simulink model "Lab_Five_QRD_Other_Input"  (R2021a)
settings: Solver=VariableStepAuto  StartTime=0.0  StopTime=double(sim_length)  RelTol=1e-3
libraries: hdlBasic x61, hdlSSR x2, xbsIndex_r4 x1
settings Model: Creator=ckk5  LastModifiedBy=ckk5

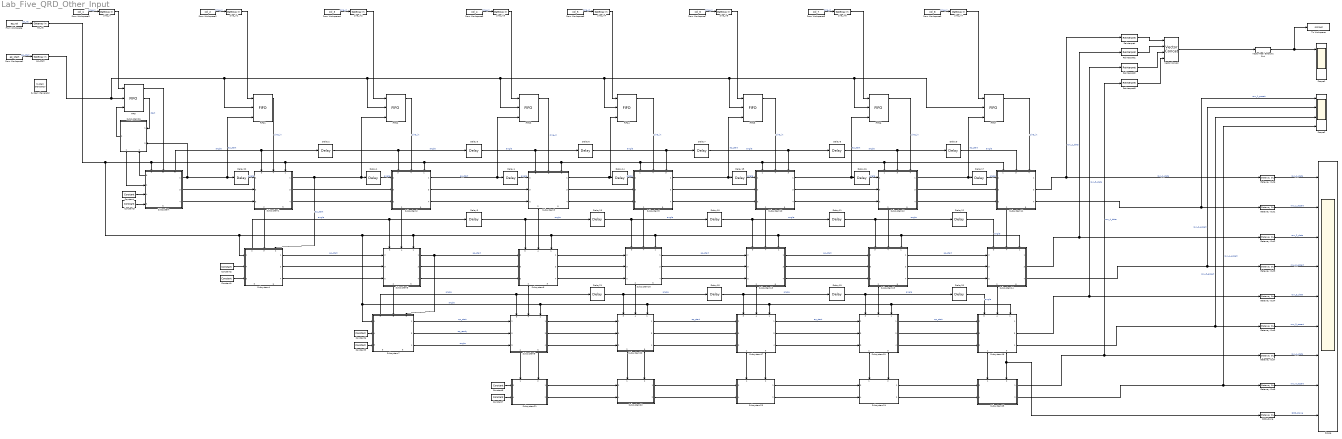
== system Lab_Five_QRD_Other_Input ==
  " System Generator" : xbsIndex_r4/ System Generator  Tag=genX  xilinxfamily=zynq  part=xc7z020  speed=-1  package=clg484  synthesis_tool=Vivado  clock_wrapper=Clock Enables  directory=./netlist  proj_type=Vivado  Synth_file=Vivado Synthesis Defaults  Impl_file=Vivado Implementation Defaults  testbench=off  simulink_period=1  sysclk_period=10  dcm_input_clock_period=10  incr_netlist=off  trim_vbits=Everywhere in SubSystem  dbl_ovrd=According to Block Masks  core_generation=According to Block Masks  run_coregen=off  deprecated_control=off  eval_field=0  block_type=sysgen
  Constant{,2,6,8} (4 alike) : hdlBasic/Constant  const=0  gui_display_data_type=Fixed-point  arith_type=Signed (2's comp)  n_bits=16  bin_pt=12  preci_type=Single  exp_width=8  frac_width=24  explicit_period=off  period=1  XmcBlockStatus=1  maskContainerNames=tabcontainer1  block_type=constant  block_config=sysgen:Constant_config
  Constant1 : hdlBasic/Constant  const=0  gui_display_data_type=Boolean  arith_type=Boolean  n_bits=16  bin_pt=12  preci_type=Single  exp_width=8  frac_width=24  explicit_period=off  period=1  XmcBlockStatus=1  maskContainerNames=tabcontainer1  block_type=constant  block_config=sysgen:Constant_config
  Constant3 : hdlBasic/Constant  const=0  gui_display_data_type=Boolean  arith_type=Boolean  n_bits=16  bin_pt=14  preci_type=Single  exp_width=8  frac_width=24  explicit_period=off  period=1  XmcBlockStatus=1  maskContainerNames=tabcontainer1  block_type=constant  block_config=sysgen:Constant_config
  Constant5 : hdlBasic/Constant  const=0  gui_display_data_type=Boolean  arith_type=Boolean  n_bits=16  bin_pt=12  preci_type=Single  exp_width=8  frac_width=24  explicit_period=off  period=1  XmcBlockStatus=1  maskContainerNames=tabcontainer1  block_type=constant  block_config=sysgen:Constant_config
  Constant7 : hdlBasic/Constant  const=0  gui_display_data_type=Boolean  arith_type=Boolean  n_bits=16  bin_pt=12  preci_type=Single  exp_width=8  frac_width=24  explicit_period=off  period=1  XmcBlockStatus=1  maskContainerNames=tabcontainer1  block_type=constant  block_config=sysgen:Constant_config
  Delay{1,4,14..17,22} (7 alike) : hdlBasic/Delay  rst=off  en=off  latency=1  reg_retiming=off  XmcBlockStatus=1  maskContainerNames=group1  block_type=delay  block_config=sysgen:Delay_config
  Delay{2..3,5..13,18..21} (15 alike) : hdlBasic/Delay  rst=off  en=off  latency=unit_L  reg_retiming=off  XmcBlockStatus=1  maskContainerNames=group1  block_type=delay  block_config=sysgen:Delay_config
  FIFO{,1..7} (8 alike) : hdlBasic/FIFO  mem_type=Block RAM  performance_options=Standard_FIFO  embedded_registers=off  depth=16  use_asym_data_widths=off  asym_read_width=32  percent_nbits=1  rst=off  rst_latency=1  en=off  use_dcount=off  use_percent_full_port=off  use_almost_empty=off  almost_empty_thresh=2  use_almost_full=off  use_rd_rst_busy=off  use_wr_rst_busy=off  almost_full_thresh=13  almost_empty_offset=[]  almost_full_offset=[]  explicit_period=off  period=[]  store_only_valid=[]  init_zero=[]  simulation_type=fast_sim  XmcBlockStatus=1  maskContainerNames=tabcontainer1  block_type=fifo  block_config=sysgen:FIFO_config
      settings: infoedit=[]
  From Workspace : FromWorkspace  VariableName=ap_rst
  From Workspace1 : FromWorkspace  VariableName=ap_start  OutputAfterFinalValue=Holding final value
  From Workspace2 : FromWorkspace  VariableName=col_2
  From Workspace3 : FromWorkspace  VariableName=col_1  OutputAfterFinalValue=Holding final value
  From Workspace4 : FromWorkspace  VariableName=col_3
  From Workspace5 : FromWorkspace  VariableName=col_4
  From Workspace6 : FromWorkspace  VariableName=col_5
  From Workspace7 : FromWorkspace  VariableName=col_6
  From Workspace8 : FromWorkspace  VariableName=col_7
  From Workspace9 : FromWorkspace  VariableName=col_8
  Gateway Out{1..8} (8 alike) : hdlBasic/Gateway Out  inherit_from_input=off  hdl_port=on  rows=1  columns=1  UseAsDAC=off  DACChannel='1'  interface=None  automatic_assignment=on  address_offset=hex2dec('00')  intf_name=''  intf_description=''  timing_constraint=None  locs_specified=off  LOCs={}  io_standard={}  XmcBlockStatus=1  maskContainerNames=group4  block_type=gatewayout  block_config=sysgen:gateway_out_config  block_width_w=590  block_height_w=620  block_width=620  block_height=750
  QRD_Done : hdlBasic/Gateway Out  inherit_from_input=off  hdl_port=on  rows=1  columns=1  UseAsDAC=off  DACChannel='1'  interface=None  automatic_assignment=on  address_offset=hex2dec('00')  intf_name=''  intf_description=''  timing_constraint=None  locs_specified=off  LOCs={}  io_standard={}  XmcBlockStatus=1  maskContainerNames=group4  block_type=gatewayout  block_config=sysgen:gateway_out_config  block_width_w=590  block_height_w=620  block_width=620  block_height=750
  Reinterpret{,1..3} (4 alike) : hdlBasic/Reinterpret  force_arith_type=on  arith_type=Unsigned  force_bin_pt=on  bin_pt=0  XmcBlockStatus=1  maskContainerNames=group1  block_type=reinterpret  block_config=sysgen:Reinterpret_config
  Scope : Scope  NumInputPorts=9
  Scope1 : Scope  NumInputPorts=3
  Scope2 : Scope  NumInputPorts=4
  Subsystem : Subsystem  ReferencedSubsystem=ATAN
      settings: PortSchema="{\"entries\":[{\"content\":{\"sides\":[{\"content\":{\"connectorIds\":[\"Out6\",\"In2\",\"In4\",\"In5\"]},\"type\":\"ConnectorPlacement.EquallySpacedRectSide\",\"uuid\":\"1346c518-8b2f-4526-a2ea-39cbeadf4b85\"},{\"content\":{\"connectorIds\":[\"Out1\",\"Out3\",\"Out4\"],\"side\":\"RIGHT\"},\"type\":\"ConnectorPlacement.EquallySpacedRectSide\",\"uuid\":\"7c1b3206-bde6-4225-9c16-bfac1b31b1ce\"},{\"content\":{\"connectorIds\":[\"In1\",\"In3\",\"Out2\"],\"side\":\"TOP\"},\"type\":\"ConnectorPlacement.EquallySpacedRectSide\",\"uuid\":\"34800851-84f6-4615-adc5-1b8c9e241528\"},{\"content\":{\"connectorIds\":[\"Out5\"],\"side\":\"BOTTOM\"},\"type\":\"ConnectorPlacement.EquallySpacedRectSide\",\"uuid\":\"52413a32-a386-4ce7-b0e4-3384f003f446\"}]},\"type\":\"ConnectorPlacement.EquallySpacedConnector\",\"uuid\":\"4bca380c-1fcc-49d9-b3a4-0ea90ddd08bc\"}],\"packageUris\":[\"http://schema.mathworks.com/mf0/Connector/R2020b\"],\"version\":\"1.0\"}"
  Subsystem{1..3,5..6,8..20} (18 alike) : Subsystem  ReferencedSubsystem=ROT
      Subsystem1 settings: PortSchema="{\"entries\":[{\"content\":{\"sides\":[{\"content\":{\"connectorIds\":[\"In2\",\"In5\",\"In6\"]},\"type\":\"ConnectorPlacement.EquallySpacedRectSide\",\"uuid\":\"c545b77a-6185-4f00-b3c2-6f0e95b73481\"},{\"content\":{\"connectorIds\":[\"Out1\",\"Out3\",\"Out4\"],\"side\":\"RIGHT\"},\"type\":\"ConnectorPlacement.EquallySpacedRectSide\",\"uuid\":\"77b30f40-c5e6-4fc5-a8bf-3f587adee46d\"},{\"content\":{\"connectorIds\":[\"In3\",\"In4\",\"In1\"],\"side\":\"TOP\"},\"type\":\"ConnectorPlacement.EquallySpacedRectSide\",\"uuid\":\"0350c9e1-b4fb-456c-83bc-c0f4f7513119\"},{\"content\":{\"connectorIds\":[\"Out2\",\"Out5\"],\"side\":\"BOTTOM\"},\"type\":\"ConnectorPlacement.EquallySpacedRectSide\",\"uuid\":\"941caaa4-bb26-4816-a397-9ab84bd5a497\"}]},\"type\":\"ConnectorPlacement.EquallySpacedConnector\",\"uuid\":\"f70f627f-f2df-4c33-aee4-d408a53254f2\"}],\"packageUris\":[\"http://schema.mathworks.com/mf0/Connector/R2020b\"],\"version\":\"1.0\"}"
      Subsystem10 settings: PortSchema="{\"entries\":[{\"content\":{\"sides\":[{\"content\":{\"connectorIds\":[\"In2\",\"In5\",\"In6\"]},\"type\":\"ConnectorPlacement.EquallySpacedRectSide\",\"uuid\":\"c545b77a-6185-4f00-b3c2-6f0e95b73481\"},{\"content\":{\"connectorIds\":[\"Out1\",\"Out3\",\"Out4\"],\"side\":\"RIGHT\"},\"type\":\"ConnectorPlacement.EquallySpacedRectSide\",\"uuid\":\"77b30f40-c5e6-4fc5-a8bf-3f587adee46d\"},{\"content\":{\"connectorIds\":[\"In1\",\"In4\",\"In3\"],\"side\":\"TOP\"},\"type\":\"ConnectorPlacement.EquallySpacedRectSide\",\"uuid\":\"0350c9e1-b4fb-456c-83bc-c0f4f7513119\"},{\"content\":{\"connectorIds\":[\"Out2\",\"Out5\"],\"side\":\"BOTTOM\"},\"type\":\"ConnectorPlacement.EquallySpacedRectSide\",\"uuid\":\"762d5bef-bc89-4a37-a25e-dba0fd023964\"}]},\"type\":\"ConnectorPlacement.EquallySpacedConnector\",\"uuid\":\"f70f627f-f2df-4c33-aee4-d408a53254f2\"}],\"packageUris\":[\"http://schema.mathworks.com/mf0/Connector/R2020b\"],\"version\":\"1.0\"}"
      Subsystem11 settings: PortSchema="{\"entries\":[{\"content\":{\"sides\":[{\"content\":{\"connectorIds\":[\"In2\",\"In5\",\"In6\"]},\"type\":\"ConnectorPlacement.EquallySpacedRectSide\",\"uuid\":\"c545b77a-6185-4f00-b3c2-6f0e95b73481\"},{\"content\":{\"connectorIds\":[\"Out1\",\"Out3\",\"Out4\"],\"side\":\"RIGHT\"},\"type\":\"ConnectorPlacement.EquallySpacedRectSide\",\"uuid\":\"77b30f40-c5e6-4fc5-a8bf-3f587adee46d\"},{\"content\":{\"connectorIds\":[\"In1\",\"In3\",\"In4\"],\"side\":\"TOP\"},\"type\":\"ConnectorPlacement.EquallySpacedRectSide\",\"uuid\":\"0350c9e1-b4fb-456c-83bc-c0f4f7513119\"},{\"content\":{\"connectorIds\":[\"Out2\",\"Out5\"],\"side\":\"BOTTOM\"},\"type\":\"ConnectorPlacement.EquallySpacedRectSide\",\"uuid\":\"5cdcca09-d0a6-4fbe-ad32-f85ef7564229\"}]},\"type\":\"ConnectorPlacement.EquallySpacedConnector\",\"uuid\":\"f70f627f-f2df-4c33-aee4-d408a53254f2\"}],\"packageUris\":[\"http://schema.mathworks.com/mf0/Connector/R2020b\"],\"version\":\"1.0\"}"
      Subsystem12 settings: PortSchema="{\"entries\":[{\"content\":{\"sides\":[{\"content\":{\"connectorIds\":[\"In2\",\"In5\",\"In6\"]},\"type\":\"ConnectorPlacement.EquallySpacedRectSide\",\"uuid\":\"c545b77a-6185-4f00-b3c2-6f0e95b73481\"},{\"content\":{\"connectorIds\":[\"Out1\",\"Out3\",\"Out4\"],\"side\":\"RIGHT\"},\"type\":\"ConnectorPlacement.EquallySpacedRectSide\",\"uuid\":\"77b30f40-c5e6-4fc5-a8bf-3f587adee46d\"},{\"content\":{\"connectorIds\":[\"In1\",\"In3\",\"In4\"],\"side\":\"TOP\"},\"type\":\"ConnectorPlacement.EquallySpacedRectSide\",\"uuid\":\"0350c9e1-b4fb-456c-83bc-c0f4f7513119\"},{\"content\":{\"connectorIds\":[\"Out2\",\"Out5\"],\"side\":\"BOTTOM\"},\"type\":\"ConnectorPlacement.EquallySpacedRectSide\",\"uuid\":\"eee39a82-822b-43a0-8e38-2b49c729ce24\"}]},\"type\":\"ConnectorPlacement.EquallySpacedConnector\",\"uuid\":\"f70f627f-f2df-4c33-aee4-d408a53254f2\"}],\"packageUris\":[\"http://schema.mathworks.com/mf0/Connector/R2020b\"],\"version\":\"1.0\"}"
      Subsystem13 settings: PortSchema="{\"entries\":[{\"content\":{\"sides\":[{\"content\":{\"connectorIds\":[\"In2\",\"In5\",\"In6\"]},\"type\":\"ConnectorPlacement.EquallySpacedRectSide\",\"uuid\":\"c545b77a-6185-4f00-b3c2-6f0e95b73481\"},{\"content\":{\"connectorIds\":[\"Out1\",\"Out3\",\"Out4\"],\"side\":\"RIGHT\"},\"type\":\"ConnectorPlacement.EquallySpacedRectSide\",\"uuid\":\"77b30f40-c5e6-4fc5-a8bf-3f587adee46d\"},{\"content\":{\"connectorIds\":[\"In3\",\"In4\",\"In1\"],\"side\":\"TOP\"},\"type\":\"ConnectorPlacement.EquallySpacedRectSide\",\"uuid\":\"0350c9e1-b4fb-456c-83bc-c0f4f7513119\"},{\"content\":{\"connectorIds\":[\"Out2\",\"Out5\"],\"side\":\"BOTTOM\"},\"type\":\"ConnectorPlacement.EquallySpacedRectSide\",\"uuid\":\"123044bf-0605-4816-88b3-d54ecb8af519\"}]},\"type\":\"ConnectorPlacement.EquallySpacedConnector\",\"uuid\":\"f70f627f-f2df-4c33-aee4-d408a53254f2\"}],\"packageUris\":[\"http://schema.mathworks.com/mf0/Connector/R2020b\"],\"version\":\"1.0\"}"
      Subsystem14 settings: PortSchema="{\"entries\":[{\"content\":{\"sides\":[{\"content\":{\"connectorIds\":[\"In2\",\"In5\",\"In6\"]},\"type\":\"ConnectorPlacement.EquallySpacedRectSide\",\"uuid\":\"c545b77a-6185-4f00-b3c2-6f0e95b73481\"},{\"content\":{\"connectorIds\":[\"Out1\",\"Out3\",\"Out4\"],\"side\":\"RIGHT\"},\"type\":\"ConnectorPlacement.EquallySpacedRectSide\",\"uuid\":\"77b30f40-c5e6-4fc5-a8bf-3f587adee46d\"},{\"content\":{\"connectorIds\":[\"In3\",\"In4\",\"In1\"],\"side\":\"TOP\"},\"type\":\"ConnectorPlacement.EquallySpacedRectSide\",\"uuid\":\"0350c9e1-b4fb-456c-83bc-c0f4f7513119\"},{\"content\":{\"connectorIds\":[\"Out2\",\"Out5\"],\"side\":\"BOTTOM\"},\"type\":\"ConnectorPlacement.EquallySpacedRectSide\",\"uuid\":\"c378bf0f-4acf-4a5e-92e8-43e03dc0127f\"}]},\"type\":\"ConnectorPlacement.EquallySpacedConnector\",\"uuid\":\"f70f627f-f2df-4c33-aee4-d408a53254f2\"}],\"packageUris\":[\"http://schema.mathworks.com/mf0/Connector/R2020b\"],\"version\":\"1.0\"}"
      Subsystem15 settings: PortSchema="{\"entries\":[{\"content\":{\"sides\":[{\"content\":{\"connectorIds\":[\"In2\",\"In5\",\"In6\"]},\"type\":\"ConnectorPlacement.EquallySpacedRectSide\",\"uuid\":\"c545b77a-6185-4f00-b3c2-6f0e95b73481\"},{\"content\":{\"connectorIds\":[\"Out1\",\"Out3\",\"Out4\"],\"side\":\"RIGHT\"},\"type\":\"ConnectorPlacement.EquallySpacedRectSide\",\"uuid\":\"77b30f40-c5e6-4fc5-a8bf-3f587adee46d\"},{\"content\":{\"connectorIds\":[\"In3\",\"In4\",\"In1\"],\"side\":\"TOP\"},\"type\":\"ConnectorPlacement.EquallySpacedRectSide\",\"uuid\":\"0350c9e1-b4fb-456c-83bc-c0f4f7513119\"},{\"content\":{\"connectorIds\":[\"Out2\",\"Out5\"],\"side\":\"BOTTOM\"},\"type\":\"ConnectorPlacement.EquallySpacedRectSide\",\"uuid\":\"d7dbbe88-442b-4e14-87a2-1b50104b2bcd\"}]},\"type\":\"ConnectorPlacement.EquallySpacedConnector\",\"uuid\":\"f70f627f-f2df-4c33-aee4-d408a53254f2\"}],\"packageUris\":[\"http://schema.mathworks.com/mf0/Connector/R2020b\"],\"version\":\"1.0\"}"
      Subsystem16 settings: PortSchema="{\"entries\":[{\"content\":{\"sides\":[{\"content\":{\"connectorIds\":[\"In2\",\"In5\",\"In6\"]},\"type\":\"ConnectorPlacement.EquallySpacedRectSide\",\"uuid\":\"c545b77a-6185-4f00-b3c2-6f0e95b73481\"},{\"content\":{\"connectorIds\":[\"Out1\",\"Out3\",\"Out4\"],\"side\":\"RIGHT\"},\"type\":\"ConnectorPlacement.EquallySpacedRectSide\",\"uuid\":\"77b30f40-c5e6-4fc5-a8bf-3f587adee46d\"},{\"content\":{\"connectorIds\":[\"In3\",\"In4\",\"In1\"],\"side\":\"TOP\"},\"type\":\"ConnectorPlacement.EquallySpacedRectSide\",\"uuid\":\"0350c9e1-b4fb-456c-83bc-c0f4f7513119\"},{\"content\":{\"connectorIds\":[\"Out2\",\"Out5\"],\"side\":\"BOTTOM\"},\"type\":\"ConnectorPlacement.EquallySpacedRectSide\",\"uuid\":\"9556fa50-b1e5-4995-ad98-fda291ad635e\"}]},\"type\":\"ConnectorPlacement.EquallySpacedConnector\",\"uuid\":\"f70f627f-f2df-4c33-aee4-d408a53254f2\"}],\"packageUris\":[\"http://schema.mathworks.com/mf0/Connector/R2020b\"],\"version\":\"1.0\"}"
      Subsystem17 settings: PortSchema="{\"entries\":[{\"content\":{\"sides\":[{\"content\":{\"connectorIds\":[\"In2\",\"In5\",\"In6\"]},\"type\":\"ConnectorPlacement.EquallySpacedRectSide\",\"uuid\":\"c545b77a-6185-4f00-b3c2-6f0e95b73481\"},{\"content\":{\"connectorIds\":[\"Out1\",\"Out3\",\"Out4\"],\"side\":\"RIGHT\"},\"type\":\"ConnectorPlacement.EquallySpacedRectSide\",\"uuid\":\"77b30f40-c5e6-4fc5-a8bf-3f587adee46d\"},{\"content\":{\"connectorIds\":[\"In3\",\"In4\",\"In1\"],\"side\":\"TOP\"},\"type\":\"ConnectorPlacement.EquallySpacedRectSide\",\"uuid\":\"0350c9e1-b4fb-456c-83bc-c0f4f7513119\"},{\"content\":{\"connectorIds\":[\"Out2\",\"Out5\"],\"side\":\"BOTTOM\"},\"type\":\"ConnectorPlacement.EquallySpacedRectSide\",\"uuid\":\"123044bf-0605-4816-88b3-d54ecb8af519\"}]},\"type\":\"ConnectorPlacement.EquallySpacedConnector\",\"uuid\":\"f70f627f-f2df-4c33-aee4-d408a53254f2\"}],\"packageUris\":[\"http://schema.mathworks.com/mf0/Connector/R2020b\"],\"version\":\"1.0\"}"
      Subsystem18 settings: PortSchema="{\"entries\":[{\"content\":{\"sides\":[{\"content\":{\"connectorIds\":[\"In2\",\"In5\",\"In6\"]},\"type\":\"ConnectorPlacement.EquallySpacedRectSide\",\"uuid\":\"c545b77a-6185-4f00-b3c2-6f0e95b73481\"},{\"content\":{\"connectorIds\":[\"Out1\",\"Out3\",\"Out4\"],\"side\":\"RIGHT\"},\"type\":\"ConnectorPlacement.EquallySpacedRectSide\",\"uuid\":\"77b30f40-c5e6-4fc5-a8bf-3f587adee46d\"},{\"content\":{\"connectorIds\":[\"In3\",\"In4\",\"In1\"],\"side\":\"TOP\"},\"type\":\"ConnectorPlacement.EquallySpacedRectSide\",\"uuid\":\"0350c9e1-b4fb-456c-83bc-c0f4f7513119\"},{\"content\":{\"connectorIds\":[\"Out2\",\"Out5\"],\"side\":\"BOTTOM\"},\"type\":\"ConnectorPlacement.EquallySpacedRectSide\",\"uuid\":\"d882beaa-ab78-4a12-aee9-70b010452786\"}]},\"type\":\"ConnectorPlacement.EquallySpacedConnector\",\"uuid\":\"f70f627f-f2df-4c33-aee4-d408a53254f2\"}],\"packageUris\":[\"http://schema.mathworks.com/mf0/Connector/R2020b\"],\"version\":\"1.0\"}"
      Subsystem19 settings: PortSchema="{\"entries\":[{\"content\":{\"sides\":[{\"content\":{\"connectorIds\":[\"In2\",\"In5\",\"In6\"]},\"type\":\"ConnectorPlacement.EquallySpacedRectSide\",\"uuid\":\"c545b77a-6185-4f00-b3c2-6f0e95b73481\"},{\"content\":{\"connectorIds\":[\"Out1\",\"Out3\",\"Out4\"],\"side\":\"RIGHT\"},\"type\":\"ConnectorPlacement.EquallySpacedRectSide\",\"uuid\":\"77b30f40-c5e6-4fc5-a8bf-3f587adee46d\"},{\"content\":{\"connectorIds\":[\"In3\",\"In4\",\"In1\"],\"side\":\"TOP\"},\"type\":\"ConnectorPlacement.EquallySpacedRectSide\",\"uuid\":\"0350c9e1-b4fb-456c-83bc-c0f4f7513119\"},{\"content\":{\"connectorIds\":[\"Out2\",\"Out5\"],\"side\":\"BOTTOM\"},\"type\":\"ConnectorPlacement.EquallySpacedRectSide\",\"uuid\":\"d7dbbe88-442b-4e14-87a2-1b50104b2bcd\"}]},\"type\":\"ConnectorPlacement.EquallySpacedConnector\",\"uuid\":\"f70f627f-f2df-4c33-aee4-d408a53254f2\"}],\"packageUris\":[\"http://schema.mathworks.com/mf0/Connector/R2020b\"],\"version\":\"1.0\"}"
      Subsystem2 settings: PortSchema="{\"entries\":[{\"content\":{\"sides\":[{\"content\":{\"connectorIds\":[\"In2\",\"In5\",\"In6\"]},\"type\":\"ConnectorPlacement.EquallySpacedRectSide\",\"uuid\":\"c545b77a-6185-4f00-b3c2-6f0e95b73481\"},{\"content\":{\"connectorIds\":[\"Out1\",\"Out3\",\"Out4\"],\"side\":\"RIGHT\"},\"type\":\"ConnectorPlacement.EquallySpacedRectSide\",\"uuid\":\"77b30f40-c5e6-4fc5-a8bf-3f587adee46d\"},{\"content\":{\"connectorIds\":[\"In3\",\"In4\",\"In1\"],\"side\":\"TOP\"},\"type\":\"ConnectorPlacement.EquallySpacedRectSide\",\"uuid\":\"0350c9e1-b4fb-456c-83bc-c0f4f7513119\"},{\"content\":{\"connectorIds\":[\"Out2\",\"Out5\"],\"side\":\"BOTTOM\"},\"type\":\"ConnectorPlacement.EquallySpacedRectSide\",\"uuid\":\"9359a6a3-4861-4aac-b9db-7dc0ab9ac5b9\"}]},\"type\":\"ConnectorPlacement.EquallySpacedConnector\",\"uuid\":\"f70f627f-f2df-4c33-aee4-d408a53254f2\"}],\"packageUris\":[\"http://schema.mathworks.com/mf0/Connector/R2020b\"],\"version\":\"1.0\"}"
      Subsystem20 settings: PortSchema="{\"entries\":[{\"content\":{\"sides\":[{\"content\":{\"connectorIds\":[\"In2\",\"In5\",\"In6\"]},\"type\":\"ConnectorPlacement.EquallySpacedRectSide\",\"uuid\":\"c545b77a-6185-4f00-b3c2-6f0e95b73481\"},{\"content\":{\"connectorIds\":[\"Out1\",\"Out3\",\"Out4\"],\"side\":\"RIGHT\"},\"type\":\"ConnectorPlacement.EquallySpacedRectSide\",\"uuid\":\"77b30f40-c5e6-4fc5-a8bf-3f587adee46d\"},{\"content\":{\"connectorIds\":[\"In3\",\"In4\",\"In1\"],\"side\":\"TOP\"},\"type\":\"ConnectorPlacement.EquallySpacedRectSide\",\"uuid\":\"0350c9e1-b4fb-456c-83bc-c0f4f7513119\"},{\"content\":{\"connectorIds\":[\"Out2\",\"Out5\"],\"side\":\"BOTTOM\"},\"type\":\"ConnectorPlacement.EquallySpacedRectSide\",\"uuid\":\"9556fa50-b1e5-4995-ad98-fda291ad635e\"}]},\"type\":\"ConnectorPlacement.EquallySpacedConnector\",\"uuid\":\"f70f627f-f2df-4c33-aee4-d408a53254f2\"}],\"packageUris\":[\"http://schema.mathworks.com/mf0/Connector/R2020b\"],\"version\":\"1.0\"}"
      Subsystem3 settings: PortSchema="{\"entries\":[{\"content\":{\"sides\":[{\"content\":{\"connectorIds\":[\"In2\",\"In5\",\"In6\"]},\"type\":\"ConnectorPlacement.EquallySpacedRectSide\",\"uuid\":\"c545b77a-6185-4f00-b3c2-6f0e95b73481\"},{\"content\":{\"connectorIds\":[\"Out1\",\"Out3\",\"Out4\"],\"side\":\"RIGHT\"},\"type\":\"ConnectorPlacement.EquallySpacedRectSide\",\"uuid\":\"77b30f40-c5e6-4fc5-a8bf-3f587adee46d\"},{\"content\":{\"connectorIds\":[\"In3\",\"In4\",\"In1\"],\"side\":\"TOP\"},\"type\":\"ConnectorPlacement.EquallySpacedRectSide\",\"uuid\":\"0350c9e1-b4fb-456c-83bc-c0f4f7513119\"},{\"content\":{\"connectorIds\":[\"Out2\",\"Out5\"],\"side\":\"BOTTOM\"},\"type\":\"ConnectorPlacement.EquallySpacedRectSide\",\"uuid\":\"8be21b47-252e-49f0-b877-01a730546064\"}]},\"type\":\"ConnectorPlacement.EquallySpacedConnector\",\"uuid\":\"f70f627f-f2df-4c33-aee4-d408a53254f2\"}],\"packageUris\":[\"http://schema.mathworks.com/mf0/Connector/R2020b\"],\"version\":\"1.0\"}"
      Subsystem5 settings: PortSchema="{\"entries\":[{\"content\":{\"sides\":[{\"content\":{\"connectorIds\":[\"In2\",\"In5\",\"In6\"]},\"type\":\"ConnectorPlacement.EquallySpacedRectSide\",\"uuid\":\"c545b77a-6185-4f00-b3c2-6f0e95b73481\"},{\"content\":{\"connectorIds\":[\"Out1\",\"Out3\",\"Out4\"],\"side\":\"RIGHT\"},\"type\":\"ConnectorPlacement.EquallySpacedRectSide\",\"uuid\":\"77b30f40-c5e6-4fc5-a8bf-3f587adee46d\"},{\"content\":{\"connectorIds\":[\"In3\",\"In4\",\"In1\"],\"side\":\"TOP\"},\"type\":\"ConnectorPlacement.EquallySpacedRectSide\",\"uuid\":\"0350c9e1-b4fb-456c-83bc-c0f4f7513119\"},{\"content\":{\"connectorIds\":[\"Out2\",\"Out5\"],\"side\":\"BOTTOM\"},\"type\":\"ConnectorPlacement.EquallySpacedRectSide\",\"uuid\":\"8ce605ee-a3e7-450c-b19e-841b4c6bf8e9\"}]},\"type\":\"ConnectorPlacement.EquallySpacedConnector\",\"uuid\":\"f70f627f-f2df-4c33-aee4-d408a53254f2\"}],\"packageUris\":[\"http://schema.mathworks.com/mf0/Connector/R2020b\"],\"version\":\"1.0\"}"
      Subsystem6 settings: PortSchema="{\"entries\":[{\"content\":{\"sides\":[{\"content\":{\"connectorIds\":[\"In2\",\"In5\",\"In6\"]},\"type\":\"ConnectorPlacement.EquallySpacedRectSide\",\"uuid\":\"c545b77a-6185-4f00-b3c2-6f0e95b73481\"},{\"content\":{\"connectorIds\":[\"Out1\",\"Out3\",\"Out4\"],\"side\":\"RIGHT\"},\"type\":\"ConnectorPlacement.EquallySpacedRectSide\",\"uuid\":\"77b30f40-c5e6-4fc5-a8bf-3f587adee46d\"},{\"content\":{\"connectorIds\":[\"In3\",\"In4\",\"In1\"],\"side\":\"TOP\"},\"type\":\"ConnectorPlacement.EquallySpacedRectSide\",\"uuid\":\"0350c9e1-b4fb-456c-83bc-c0f4f7513119\"},{\"content\":{\"connectorIds\":[\"Out2\",\"Out5\"],\"side\":\"BOTTOM\"},\"type\":\"ConnectorPlacement.EquallySpacedRectSide\",\"uuid\":\"67ba7c68-e424-4a03-8b18-e6ace04697e3\"}]},\"type\":\"ConnectorPlacement.EquallySpacedConnector\",\"uuid\":\"f70f627f-f2df-4c33-aee4-d408a53254f2\"}],\"packageUris\":[\"http://schema.mathworks.com/mf0/Connector/R2020b\"],\"version\":\"1.0\"}"
      Subsystem8 settings: PortSchema="{\"entries\":[{\"content\":{\"sides\":[{\"content\":{\"connectorIds\":[\"In2\",\"In5\",\"In6\"]},\"type\":\"ConnectorPlacement.EquallySpacedRectSide\",\"uuid\":\"c545b77a-6185-4f00-b3c2-6f0e95b73481\"},{\"content\":{\"connectorIds\":[\"Out1\",\"Out3\",\"Out4\"],\"side\":\"RIGHT\"},\"type\":\"ConnectorPlacement.EquallySpacedRectSide\",\"uuid\":\"77b30f40-c5e6-4fc5-a8bf-3f587adee46d\"},{\"content\":{\"connectorIds\":[\"In3\",\"In4\",\"In1\"],\"side\":\"TOP\"},\"type\":\"ConnectorPlacement.EquallySpacedRectSide\",\"uuid\":\"0350c9e1-b4fb-456c-83bc-c0f4f7513119\"},{\"content\":{\"connectorIds\":[\"Out2\",\"Out5\"],\"side\":\"BOTTOM\"},\"type\":\"ConnectorPlacement.EquallySpacedRectSide\",\"uuid\":\"3a67377a-ede4-4ab7-b2be-c5c6267492fe\"}]},\"type\":\"ConnectorPlacement.EquallySpacedConnector\",\"uuid\":\"f70f627f-f2df-4c33-aee4-d408a53254f2\"}],\"packageUris\":[\"http://schema.mathworks.com/mf0/Connector/R2020b\"],\"version\":\"1.0\"}"
      Subsystem9 settings: PortSchema="{\"entries\":[{\"content\":{\"sides\":[{\"content\":{\"connectorIds\":[\"In2\",\"In5\",\"In6\"]},\"type\":\"ConnectorPlacement.EquallySpacedRectSide\",\"uuid\":\"c545b77a-6185-4f00-b3c2-6f0e95b73481\"},{\"content\":{\"connectorIds\":[\"Out1\",\"Out3\",\"Out4\"],\"side\":\"RIGHT\"},\"type\":\"ConnectorPlacement.EquallySpacedRectSide\",\"uuid\":\"77b30f40-c5e6-4fc5-a8bf-3f587adee46d\"},{\"content\":{\"connectorIds\":[\"In1\",\"In4\",\"In3\"],\"side\":\"TOP\"},\"type\":\"ConnectorPlacement.EquallySpacedRectSide\",\"uuid\":\"0350c9e1-b4fb-456c-83bc-c0f4f7513119\"},{\"content\":{\"connectorIds\":[\"Out2\",\"Out5\"],\"side\":\"BOTTOM\"},\"type\":\"ConnectorPlacement.EquallySpacedRectSide\",\"uuid\":\"bdd32112-8c69-4693-8927-a15fce0e358b\"}]},\"type\":\"ConnectorPlacement.EquallySpacedConnector\",\"uuid\":\"f70f627f-f2df-4c33-aee4-d408a53254f2\"}],\"packageUris\":[\"http://schema.mathworks.com/mf0/Connector/R2020b\"],\"version\":\"1.0\"}"
  Subsystem{21..25} (5 alike) : Subsystem  ReferencedSubsystem=Output_Selector_Simple
      settings: PortSchema="{\"entries\":[{\"content\":{\"sides\":[{\"content\":{\"connectorIds\":[\"In3\",\"In4\"]},\"type\":\"ConnectorPlacement.EquallySpacedRectSide\",\"uuid\":\"faf72d46-e9ca-4554-a625-ae2ca42b272c\"},{\"content\":{\"connectorIds\":[\"Out1\",\"Out2\"],\"side\":\"RIGHT\"},\"type\":\"ConnectorPlacement.EquallySpacedRectSide\",\"uuid\":\"48df0ee7-6269-49be-b825-f5ec50cf44de\"},{\"content\":{\"connectorIds\":[\"In1\",\"In2\"],\"side\":\"TOP\"},\"type\":\"ConnectorPlacement.EquallySpacedRectSide\",\"uuid\":\"7b6bacea-9321-4917-b98a-2a491d68cf09\"}]},\"type\":\"ConnectorPlacement.EquallySpacedConnector\",\"uuid\":\"b4ec3097-cb8d-4869-bae0-774e19390046\"}],\"packageUris\":[\"http://schema.mathworks.com/mf0/Connector/R2020b\"],\"version\":\"1.0\"}"
  Subsystem26 : Subsystem  ReferencedSubsystem=Start_Logic_Block
      settings: PortSchema="{\"entries\":[{\"content\":{\"sides\":[{\"content\":{\"connectorIds\":[\"Out2\"]},\"type\":\"ConnectorPlacement.EquallySpacedRectSide\",\"uuid\":\"854bddad-7798-4bde-aef6-f525d1b9c2d2\"},{\"content\":{\"connectorIds\":[\"In1\",\"In3\"],\"side\":\"RIGHT\"},\"type\":\"ConnectorPlacement.EquallySpacedRectSide\",\"uuid\":\"2663665e-ec1e-43c0-abf8-99d2507509af\"},{\"content\":{\"connectorIds\":[],\"side\":\"TOP\"},\"type\":\"ConnectorPlacement.EquallySpacedRectSide\",\"uuid\":\"b225d888-10fa-4460-a1b4-18b11f556bd1\"},{\"content\":{\"connectorIds\":[\"Out1\",\"In2\"],\"side\":\"BOTTOM\"},\"type\":\"ConnectorPlacement.EquallySpacedRectSide\",\"uuid\":\"9e401118-deda-4600-a7b8-34d1b1ab15f0\"}]},\"type\":\"ConnectorPlacement.EquallySpacedConnector\",\"uuid\":\"707e5c98-5f7e-4e96-88dd-3258b4b39c7e\"}],\"packageUris\":[\"http://schema.mathworks.com/mf0/Connector/R2020b\"],\"version\":\"1.0\"}"
  Subsystem4 : Subsystem  ReferencedSubsystem=ATAN
      settings: PortSchema="{\"entries\":[{\"content\":{\"sides\":[{\"content\":{\"connectorIds\":[\"In1\",\"In4\",\"In5\"]},\"type\":\"ConnectorPlacement.EquallySpacedRectSide\",\"uuid\":\"2ab3b1c3-ccaa-47c6-871d-fe42e2674163\"},{\"content\":{\"connectorIds\":[\"Out1\",\"Out3\",\"Out4\"],\"side\":\"RIGHT\"},\"type\":\"ConnectorPlacement.EquallySpacedRectSide\",\"uuid\":\"31fb9cc9-97aa-4ac6-b8a6-a5ac9c63e2b7\"},{\"content\":{\"connectorIds\":[\"Out2\",\"In3\",\"In2\"],\"side\":\"TOP\"},\"type\":\"ConnectorPlacement.EquallySpacedRectSide\",\"uuid\":\"8eeeea61-cf7b-46f0-8c7b-badeddc1c862\"},{\"content\":{\"connectorIds\":[\"Out5\",\"Out6\"],\"side\":\"BOTTOM\"},\"type\":\"ConnectorPlacement.EquallySpacedRectSide\",\"uuid\":\"d604f620-ecbf-4849-a6ed-8f1ac529d2ef\"}]},\"type\":\"ConnectorPlacement.EquallySpacedConnector\",\"uuid\":\"282736d9-3194-4aa4-b418-8df4df1c8027\"}],\"packageUris\":[\"http://schema.mathworks.com/mf0/Connector/R2020b\"],\"version\":\"1.0\"}"
  Subsystem7 : Subsystem  ReferencedSubsystem=ATAN
      settings: PortSchema="{\"entries\":[{\"content\":{\"sides\":[{\"content\":{\"connectorIds\":[\"In1\",\"In4\",\"In5\"]},\"type\":\"ConnectorPlacement.EquallySpacedRectSide\",\"uuid\":\"2ab3b1c3-ccaa-47c6-871d-fe42e2674163\"},{\"content\":{\"connectorIds\":[\"Out1\",\"Out3\",\"Out4\"],\"side\":\"RIGHT\"},\"type\":\"ConnectorPlacement.EquallySpacedRectSide\",\"uuid\":\"31fb9cc9-97aa-4ac6-b8a6-a5ac9c63e2b7\"},{\"content\":{\"connectorIds\":[\"Out2\",\"In3\",\"In2\"],\"side\":\"TOP\"},\"type\":\"ConnectorPlacement.EquallySpacedRectSide\",\"uuid\":\"8eeeea61-cf7b-46f0-8c7b-badeddc1c862\"},{\"content\":{\"connectorIds\":[\"Out5\",\"Out6\"],\"side\":\"BOTTOM\"},\"type\":\"ConnectorPlacement.EquallySpacedRectSide\",\"uuid\":\"ad6f459e-c774-479a-8ac6-2f1de5f02012\"}]},\"type\":\"ConnectorPlacement.EquallySpacedConnector\",\"uuid\":\"282736d9-3194-4aa4-b418-8df4df1c8027\"}],\"packageUris\":[\"http://schema.mathworks.com/mf0/Connector/R2020b\"],\"version\":\"1.0\"}"
  To Workspace : ToWorkspace  VariableName=simout  SaveFormat=Structure With Time  SampleTime=-1
  Vector Concat : hdlSSR/Vector Concat  num_inputs=4  sg_ssr=1  num_inputs_prev=4  block_type=concat_ssr  XmcBlockStatus=1  sg_ssr_prev=1  maskContainerNames=group1
  Vector Real Gateway Out : hdlSSR/Vector Real Gateway Out  inherit_from_input=off  hdl_port=on  sg_ssr=1  rows=1  columns=1  UseAsDAC=off  DACChannel='1'  interface=None  automatic_assignment=on  address_offset=hex2dec('00')  intf_name=''  intf_description=''  timing_constraint=None  locs_specified=off  LOCs={}  io_standard={}  block_type=realgatewayout_ssr  XmcBlockStatus=1  sg_ssr_prev=1  maskContainerNames=group4  block_width_w=590  block_height_w=620  block_width=620  block_height=750
  ap_rst : hdlBasic/Gateway In  gui_display_data_type=Boolean  arith_type=Boolean  n_bits=16  bin_pt=14  preci_type=Single  exp_width=8  frac_width=24  rows=1  columns=1  quantization="Round  (unbiased: +/- Inf)"  overflow=Saturate  period=1  UseAsADC=off  ADCChannel='1'  interface=None  automatic_assignment=on  address_offset=hex2dec('00')  intf_name=''  intf_description=''  default_value=0  timing_constraint=None  locs_specified=off  LOCs={}  io_standard={}  inherit_from_input=off  hdl_port=on  XmcBlockStatus=1  maskContainerNames=group4  block_type=gatewayin  block_config=sysgen:gateway_in_config  block_width_w=590  block_height_w=620  block_width=640  block_height=850
  ap_start : hdlBasic/Gateway In  gui_display_data_type=Boolean  arith_type=Boolean  n_bits=16  bin_pt=14  preci_type=Single  exp_width=8  frac_width=24  rows=1  columns=1  quantization="Round  (unbiased: +/- Inf)"  overflow=Saturate  period=1  UseAsADC=off  ADCChannel='1'  interface=None  automatic_assignment=on  address_offset=hex2dec('00')  intf_name=''  intf_description=''  default_value=0  timing_constraint=None  locs_specified=off  LOCs={}  io_standard={}  inherit_from_input=off  hdl_port=on  XmcBlockStatus=1  maskContainerNames=group4  block_type=gatewayin  block_config=sysgen:gateway_in_config  block_width_w=590  block_height_w=620  block_width=640  block_height=850
  sine_in{,1..7} (8 alike) : hdlBasic/Gateway In  gui_display_data_type=Fixed-point  arith_type=Signed (2's comp)  n_bits=16  bin_pt=12  preci_type=Single  exp_width=8  frac_width=24  rows=1  columns=1  quantization="Round  (unbiased: +/- Inf)"  overflow=Saturate  period=1  UseAsADC=off  ADCChannel='1'  interface=None  automatic_assignment=on  address_offset=hex2dec('00')  intf_name=''  intf_description=''  default_value=0  timing_constraint=None  locs_specified=off  LOCs={}  io_standard={}  inherit_from_input=off  hdl_port=on  XmcBlockStatus=1  maskContainerNames=group4  block_type=gatewayin  block_config=sysgen:gateway_in_config  block_width_w=590  block_height_w=620  block_width=640  block_height=850
  wires:
  From Workspace/1 -> ap_rst/1  "ap_rst"
  From Workspace1/1 -> ap_start/1  "ap_start"
  From Workspace3/1 -> sine_in/1  "sine_in"
  Subsystem/1 -> Delay22/1, FIFO1/3, Subsystem26/3  "ap_start"
  Subsystem/2 -> Subsystem1/3, Delay2/1  "angle"
  From Workspace2/1 -> sine_in1/1  "sine_in"
  sine_in1/1 -> FIFO1/1
  FIFO1/1 -> Subsystem1/4  "sine_in"
  From Workspace4/1 -> sine_in2/1  "sine_in"
  sine_in2/1 -> FIFO2/1
  sine_in3/1 -> FIFO3/1
  From Workspace5/1 -> sine_in3/1  "sine_in"
  Delay2/1 -> Subsystem2/3, Delay3/1  "angle"
  FIFO2/1 -> Subsystem2/4  "sine_in"
  Subsystem1/1 -> FIFO2/3, Delay1/1, Subsystem4/2  "ap_start"
  FIFO3/1 -> Subsystem3/4  "sine_in"
  Subsystem2/1 -> FIFO3/3, Delay4/1  "ap_start"
  Subsystem4/1 -> Subsystem5/2  "ap_start"
  Subsystem4/2 -> Delay5/1, Subsystem5/3  "angle"
  Delay5/1 -> Delay13/1, Subsystem6/3  "angle"
  Subsystem5/1 -> Subsystem7/2, Subsystem6/2  "ap_start"
  sine_in/1 -> FIFO/1
  Subsystem7/1 -> Subsystem8/2  "ap_start"
  Delay6/1 -> Subsystem9/3, Delay7/1  "angle"
  Delay3/1 -> Subsystem3/3, Delay6/1  "angle"
  Subsystem3/1 -> FIFO4/3, Delay14/1
  Delay7/1 -> Subsystem10/3, Delay8/1  "angle"
  Delay8/1 -> Subsystem12/3, Delay9/1  "angle"
  Delay9/1 -> Subsystem11/3  "angle"
  Subsystem9/1 -> FIFO5/3, Delay15/1  "ap_start"
  Subsystem10/1 -> FIFO6/3, Delay16/1  "ap_start"
  Subsystem12/1 -> FIFO7/3, Delay17/1  "ap_start"
  Subsystem16/1 -> Subsystem13/2  "ap_start"
  Delay12/1 -> Subsystem14/3  "angle"
  Subsystem15/1 -> Subsystem14/2  "ap_start"
  Subsystem13/1 -> Subsystem15/2  "ap_start"
  Delay11/1 -> Delay12/1, Subsystem15/3  "angle"
  Subsystem6/1 -> Subsystem16/2
  Delay10/1 -> Delay11/1, Subsystem13/3  "angle"
  Delay13/1 -> Delay10/1, Subsystem16/3  "angle"
  From Workspace6/1 -> sine_in4/1  "sine_in"
  sine_in4/1 -> FIFO4/1
  FIFO4/1 -> Subsystem9/4  "sine_in"
  sine_in5/1 -> FIFO5/1
  From Workspace7/1 -> sine_in5/1  "sine_in"
  FIFO5/1 -> Subsystem10/4  "sine_in"
  sine_in6/1 -> FIFO6/1
  From Workspace8/1 -> sine_in6/1  "sine_in"
  FIFO6/1 -> Subsystem12/4  "sine_in"
  sine_in7/1 -> FIFO7/1
  From Workspace9/1 -> sine_in7/1  "sine_in"
  FIFO7/1 -> Subsystem11/4  "sine_in"
  Subsystem/3 -> Subsystem1/5
  Subsystem/4 -> Subsystem1/6
  Subsystem1/3 -> Subsystem2/5
  Subsystem1/4 -> Subsystem2/6
  Subsystem15/3 -> Subsystem14/5
  Subsystem15/4 -> Subsystem14/6
  Subsystem13/3 -> Subsystem15/5
  Subsystem13/4 -> Subsystem15/6
  Subsystem16/3 -> Subsystem13/5
  Subsystem16/4 -> Subsystem13/6
  Subsystem4/3 -> Subsystem5/5
  Subsystem4/4 -> Subsystem5/6
  Constant3/1 -> Subsystem/5
  Constant/1 -> Subsystem/4
  Subsystem10/4 -> Subsystem12/6
  Subsystem2/3 -> Subsystem3/5
  Subsystem2/4 -> Subsystem3/6
  Subsystem10/3 -> Subsystem12/5
  Subsystem12/3 -> Subsystem11/5
  Subsystem12/4 -> Subsystem11/6
  Subsystem11/2 -> Subsystem14/4
  Subsystem12/2 -> Subsystem15/4
  Subsystem10/2 -> Subsystem13/4
  Subsystem9/2 -> Subsystem16/4
  Subsystem6/3 -> Subsystem16/5
  Subsystem6/4 -> Subsystem16/6
  Subsystem6/2 -> Subsystem8/4
  Subsystem5/3 -> Subsystem6/5
  Subsystem5/4 -> Subsystem6/6
  Subsystem5/2 -> Subsystem7/3
  Subsystem3/3 -> Subsystem9/5
  Subsystem3/4 -> Subsystem9/6
  Subsystem3/2 -> Subsystem6/4
  Subsystem2/2 -> Subsystem5/4
  Constant6/1 -> Subsystem7/4
  Constant5/1 -> Subsystem7/5
  Subsystem7/3 -> Subsystem8/5  "ap_ready"
  Subsystem7/4 -> Subsystem8/6  "angle"
  Subsystem8/3 -> Subsystem20/5
  Subsystem19/3 -> Subsystem18/5
  Subsystem20/3 -> Subsystem17/5
  Subsystem13/2 -> Subsystem17/4
  Delay21/1 -> Delay18/1, Subsystem20/3  "angle"
  Subsystem8/4 -> Subsystem20/6
  Delay19/1 -> Delay20/1, Subsystem19/3  "angle"
  Subsystem15/2 -> Subsystem19/4
  Subsystem14/2 -> Subsystem18/4
  Subsystem20/4 -> Subsystem17/6
  Subsystem17/3 -> Subsystem19/5
  Subsystem19/4 -> Subsystem18/6
  Subsystem17/1 -> Subsystem19/2  "ap_start"
  Subsystem20/1 -> Subsystem17/2  "ap_start"
  Delay20/1 -> Subsystem18/3  "angle"
  Delay18/1 -> Delay19/1, Subsystem17/3  "angle"
  Subsystem7/2 -> Delay21/1, Subsystem8/3  "angle"
  Subsystem8/1 -> Subsystem20/2
  Subsystem17/4 -> Subsystem19/6
  Subsystem19/1 -> Subsystem18/2  "ap_start"
  Subsystem16/2 -> Subsystem20/4
  ap_rst/1 -> Subsystem10/1, Subsystem12/1, Subsystem11/1, Subsystem9/1, Subsystem3/1, Subsystem2/1, Subsystem1/1, Subsystem/1, Subsystem18/1, Subsystem19/1, Subsystem17/1, Subsystem20/1, Subsystem8/1, Subsystem7/1, Subsystem14/1, Subsystem15/1, Subsystem13/1, Subsystem16/1, Subsystem6/1, Subsystem5/1, Subsystem4/1  "angle"
  Subsystem9/3 -> Subsystem10/5
  Subsystem9/4 -> Subsystem10/6
  Subsystem11/3 -> Gateway Out6/1, Reinterpret/1  "row_1_data"
  Subsystem11/4 -> Scope2/1, Gateway Out1/1  "row_1_assert"
  Subsystem14/3 -> Gateway Out2/1, Reinterpret1/1  "row_2_data"
  Subsystem14/4 -> Gateway Out3/1, Scope2/2  "row_2_assert"
  Subsystem18/3 -> Gateway Out4/1, Reinterpret2/1  "row_3_data"
  Subsystem18/4 -> Scope2/3, Gateway Out5/1  "row_3_assert"
  Subsystem8/2 -> Subsystem21/1
  Subsystem8/5 -> Subsystem21/2
  Constant8/1 -> Subsystem21/3
  Constant7/1 -> Subsystem21/4
  Subsystem21/1 -> Subsystem22/3
  Subsystem21/2 -> Subsystem22/4
  Subsystem22/1 -> Subsystem23/3
  Subsystem22/2 -> Subsystem23/4
  Subsystem23/1 -> Subsystem24/3
  Subsystem23/2 -> Subsystem24/4
  Subsystem24/1 -> Subsystem25/3
  Subsystem24/2 -> Subsystem25/4
  Subsystem25/1 -> Reinterpret3/1, Gateway Out7/1  "row_4_data"
  Subsystem25/2 -> Gateway Out8/1, Scope2/4  "row_4_assert"
  Subsystem18/5 -> QRD_Done/1, Subsystem25/2
  Subsystem18/2 -> Subsystem25/1
  Subsystem19/5 -> Subsystem24/2
  Subsystem19/2 -> Subsystem24/1
  Subsystem17/5 -> Subsystem23/2
  Subsystem17/2 -> Subsystem23/1
  Subsystem20/5 -> Subsystem22/2
  Subsystem20/2 -> Subsystem22/1
  Gateway Out2/1 -> Scope/3  "row_2_data"
  Gateway Out3/1 -> Scope/4  "row_2_assert"
  Gateway Out4/1 -> Scope/5  "row_3_data"
  Gateway Out5/1 -> Scope/6  "row_3_assert"
  Gateway Out7/1 -> Scope/7  "row_4_data"
  Gateway Out8/1 -> Scope/8  "row_4_assert"
  QRD_Done/1 -> Scope/9  "QRD_Done"
  Gateway Out6/1 -> Scope/1  "row_1_data"
  Gateway Out1/1 -> Scope/2  "row_1_assert"
  Vector Concat/1 -> Vector Real Gateway Out/1
  Reinterpret/1 -> Vector Concat/1
  Reinterpret1/1 -> Vector Concat/2
  Vector Real Gateway Out/1 -> To Workspace/1, Scope1/1
  Reinterpret2/1 -> Vector Concat/3
  Reinterpret3/1 -> Vector Concat/4
  ap_start/1 -> FIFO/2, FIFO1/2, FIFO3/2, FIFO4/2, FIFO5/2, FIFO6/2, FIFO7/2, FIFO2/2
  Subsystem1/2 -> Subsystem4/3
  Constant2/1 -> Subsystem4/4
  Constant1/1 -> Subsystem4/5
  Subsystem26/1 -> Subsystem/2
  Subsystem26/2 -> FIFO/3
  FIFO/2 -> Subsystem26/1  "start"
  FIFO/1 -> Subsystem/3
  Subsystem/6 -> Subsystem26/2
  Delay22/1 -> Subsystem1/2  "angle"
  Delay1/1 -> Subsystem2/2  "angle"
  Delay4/1 -> Subsystem3/2  "angle"
  Delay14/1 -> Subsystem9/2  "angle"
  Delay15/1 -> Subsystem10/2  "angle"
  Delay16/1 -> Subsystem12/2  "angle"
  Delay17/1 -> Subsystem11/2  "angle"
